simulink model "hexapod_LC"  (R2020b)
settings: Solver=VariableStepAuto  StartTime=0.0  StopTime=40.0  RelTol=1e-3
values from neighbouring files (symbols this model uses):
  goalPose = [13 13 0]    [Run_Sim_LC.m]
  N = size(waypoints, 1)    [interpolate_leg_waypoints.m]
  startPose = [2 2 0]    [Run_Sim_LC.m]
  Ts = 0.01    [Run_Sim_LC.m]
undefined symbols (not defined in the file or in its folder): Discrete, q, qd, Time, X, Y, Z
libraries: sm_lib x12, legs x8, nesl_utility x3, robotics_pg_exp_pack x2, ctrlSharedLib x1
settings Model: Creator=fciriell  LastModifiedBy=zach
settings ExplorerConfigSet: InternalSimMechanicsExplorerSettings="<ExplorerConfiguration><canonicalview>default</canonicalview><AnimationSetting><BasePlaybackSpeed>1.0</BasePlaybackSpeed><PlaybackSpeedFactor>1.0</PlaybackSpeedFactor></AnimationSetting><TilePanel><TileInfo><Tiles Columns=\"1\" Count=\"2\" Rows=\"2\"><Column Weight=\"1\"/><Row Weight=\"0.4993\"/><Row Weight=\"0.5007\"/><Tile Height=\"1\" Width=\"1\" X=\"0\" Y=\"0\"/><Tile Height=\"1\" Width=\"1\" X=\"0\" Y=\"1\"/></Tiles></TileInfo><SceneInfo><SceneViewer><BGColor><R>1</R><G>1</G><B>1</B></BGColor><Camera><DoPerspective>on</DoPerspective><Position><X>-4.35147948962821829e-06</X><Y>-4.89869399804638128</Y><Z>0.176731420553238427</Z></Position><Center><X>-4.35147948962821829e-06</X><Y>-1.26250265135058726</Y><Z>0.176731420553238427</Z></Center><Up><X>0</X><Y>-0</Y><Z>1</Z></Up><ViewLimDist>1</ViewLimDist><YLim>0.466307658154998583</YLim><XLim>1.59125758717581123</XLim></Camera></SceneViewer><SceneViewer><BGColor><R>1</R><G>1</G><B>1</B></BGColor><Camera><DoPerspective>off</DoPerspective><Position><X>-5.9945065800093289e-08</X><Y>-3.21515629578642415</Y><Z>0.0606596897011122405</Z></Position><Center><X>-5.9945065800093289e-08</X><Y>-1.26250000733898382</Y><Z>0.0606596897011122405</Z></Center><Up><X>-0</X><Y>0</Y><Z>1</Z></Up><ViewLimDist>1</ViewLimDist><YLim>0.993270539045333911</YLim><XLim>3.37947076894122489</XLim></Camera></SceneViewer></SceneInfo></TilePanel><MechEditorPanel><Cameras><Camera><Id>Camera1</Id><Value><Name>Camera1</Name><NativeCamera><PositionTrackingFeature>camera.F</PositionTrackingFeature><CenterTrackingFeature>One_link_chain_dynamic.to_WF</CenterTrackingFeature><UpVectorTrackingFeature>camera.F</UpVectorTrackingFeature><CenterTrackingOrigin>on</CenterTrackingOrigin><UpVectorTrackingDirection>+Z</UpVectorTrackingDirection></NativeCamera></Value></Camera></Cameras><GfxPanelCameraMap><MapElement CameraMLId=\"Camera1\" GfxPanelIndex=\"0\"/></GfxPanelCameraMap><VideoCreator><PlaybackSpeedRatio>1.0</PlaybackSpeedRatio><FrameRate>30</FrameRate><VideoFormat>Motion JPEG AVI</VideoFormat><FrameSize>auto</FrameSize></VideoCreator></MechEditorPanel></ExplorerConfiguration>"

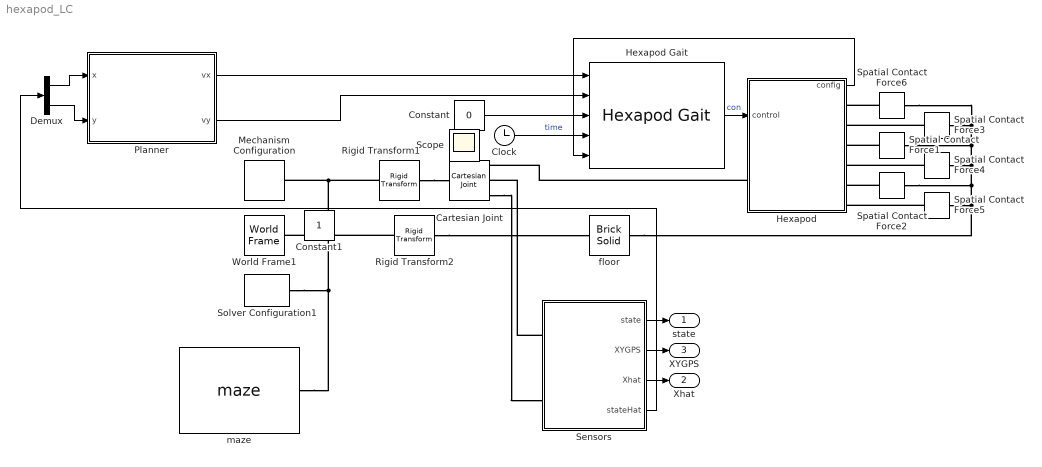
== system hexapod_LC ==
  Cartesian Joint : sm_lib/Joints/Cartesian Joint  JointMode=Normal  SenseConstraintForce=off  SenseConstraintForceX=off  SenseConstraintForceY=off  SenseConstraintForceZ=off  SenseConstraintTorque=off  SenseConstraintTorqueX=off  SenseConstraintTorqueY=off  SenseConstraintTorqueZ=off  SenseTotalForce=off  SenseTotalForceX=off  SenseTotalForceY=off  SenseTotalForceZ=off  SenseTotalTorque=off  SenseTotalTorqueX=off  SenseTotalTorqueY=off  SenseTotalTorqueZ=off  CompositeWrenchDir=FollowerOnBase  CompositeWrenchFrame=BaseFrame  PxEquilibriumPosition=0  PxEquilibriumPositionUnits=m  PxSpringStiffness=0  PxSpringStiffnessUnits=N/m  PxDampingCoefficient=0  PxDampingCoefficientUnits=N/(m/s)  PxTorqueActuationMode=NoTorque  PxMotionActuationMode=ComputedMotion  PxSensePosition=on  PxSenseVelocity=off  PxSenseAcceleration=off  PxSenseTorqueForce=off  PxSenseLowerLimitTorqueForce=off  PxSenseUpperLimitTorqueForce=off  PxLowerLimitSpecify=off  PxLowerLimitBound=-1  PxLowerLimitBoundUnits=m  PxLowerLimitStiffness=1e6  PxLowerLimitStiffnessUnits=N/m  PxLowerLimitDamping=1e3  PxLowerLimitDampingUnits=N/(m/s)  PxLowerLimitTransitionRegionWidth=1e-4  PxLowerLimitTransitionRegionWidthUnits=m  PxUpperLimitSpecify=off  PxUpperLimitBound=1  PxUpperLimitBoundUnits=m  PxUpperLimitStiffness=1e6  PxUpperLimitStiffnessUnits=N/m  PxUpperLimitDamping=1e3  PxUpperLimitDampingUnits=N/(m/s)  PxUpperLimitTransitionRegionWidth=1e-4  PxUpperLimitTransitionRegionWidthUnits=m  PxPositionTargetSpecify=on  PxPositionTargetPriority=High  PxPositionTargetValue=0  PxPositionTargetValueUnits=m  PxVelocityTargetSpecify=off  PxVelocityTargetPriority=High  PxVelocityTargetValue=0  PxVelocityTargetValueUnits=m/s  PyEquilibriumPosition=0  PyEquilibriumPositionUnits=m  PySpringStiffness=0  PySpringStiffnessUnits=N/m  PyDampingCoefficient=0  PyDampingCoefficientUnits=N/(m/s)  PyTorqueActuationMode=NoTorque  PyMotionActuationMode=ComputedMotion  PySensePosition=on  PySenseVelocity=off  PySenseAcceleration=off  PySenseTorqueForce=off  PySenseLowerLimitTorqueForce=off  PySenseUpperLimitTorqueForce=off  PyLowerLimitSpecify=off  PyLowerLimitBound=-1  PyLowerLimitBoundUnits=m  PyLowerLimitStiffness=1e6  PyLowerLimitStiffnessUnits=N/m  PyLowerLimitDamping=1e3  PyLowerLimitDampingUnits=N/(m/s)  PyLowerLimitTransitionRegionWidth=1e-4  PyLowerLimitTransitionRegionWidthUnits=m  PyUpperLimitSpecify=off  PyUpperLimitBound=1  PyUpperLimitBoundUnits=m  PyUpperLimitStiffness=1e6  PyUpperLimitStiffnessUnits=N/m  PyUpperLimitDamping=1e3  PyUpperLimitDampingUnits=N/(m/s)  PyUpperLimitTransitionRegionWidth=1e-4  PyUpperLimitTransitionRegionWidthUnits=m  PyPositionTargetSpecify=on  PyPositionTargetPriority=High  PyPositionTargetValue=0  PyPositionTargetValueUnits=m  PyVelocityTargetSpecify=off  PyVelocityTargetPriority=High  PyVelocityTargetValue=0  PyVelocityTargetValueUnits=m/s  PzEquilibriumPosition=0  PzEquilibriumPositionUnits=m  PzSpringStiffness=0  PzSpringStiffnessUnits=N/m  PzDampingCoefficient=0  PzDampingCoefficientUnits=N/(m/s)  PzTorqueActuationMode=NoTorque  PzMotionActuationMode=ComputedMotion  PzSensePosition=off  PzSenseVelocity=off  PzSenseAcceleration=off  PzSenseTorqueForce=off  PzSenseLowerLimitTorqueForce=off  PzSenseUpperLimitTorqueForce=off  PzLowerLimitSpecify=off  PzLowerLimitBound=-1  PzLowerLimitBoundUnits=m  PzLowerLimitStiffness=1e6  PzLowerLimitStiffnessUnits=N/m  PzLowerLimitDamping=1e3  PzLowerLimitDampingUnits=N/(m/s)  PzLowerLimitTransitionRegionWidth=1e-4  PzLowerLimitTransitionRegionWidthUnits=m  PzUpperLimitSpecify=off  PzUpperLimitBound=1  PzUpperLimitBoundUnits=m  PzUpperLimitStiffness=1e6  PzUpperLimitStiffnessUnits=N/m  PzUpperLimitDamping=1e3  PzUpperLimitDampingUnits=N/(m/s)  PzUpperLimitTransitionRegionWidth=1e-4  PzUpperLimitTransitionRegionWidthUnits=m  PzPositionTargetSpecify=on  PzPositionTargetPriority=High  PzPositionTargetValue=0.6  PzPositionTargetValueUnits=m  PzVelocityTargetSpecify=off  PzVelocityTargetPriority=High  PzVelocityTargetValue=0  PzVelocityTargetValueUnits=m/s
  Clock : Clock
  Constant : Constant  Value=0  SampleTime=-1
  Demux : Demux  Outputs=2
  Hexapod : Subsystem  AncestorBlock=legs/Hexapod  mask{leg_initial_config=[0; pi/8; 3*pi/8], leg_length_1=0.1, leg_length_2=0.4, leg_length_3=0.4, leg_radius=0.04, leg_mass_1=0.1, leg_mass_2=0.3, leg_mass_3=0.3, pos_kp=[40; 40; 40], pos_ki=[0; 0; 0], pos_kd=[4; 4; 4], body_radius=0.3, body_mass=0.2}
      mask prompts: leg_initial_config "Leg initial config"; leg_length_1 "Leg length 1"; leg_length_2 "Leg length 2"; leg_length_3 "Leg length 3"; leg_radius "Leg radius"; leg_mass_1 "Leg mass 1"; leg_mass_2 "Leg mass 2"; leg_mass_3 "Leg mass 3"; pos_kp "Position control kp"; pos_ki "Position control ki"; pos_kd "Position control kd"; body_radius "Body radius"; body_mass "Body mass"
  Hexapod Gait : legs/Hexapod Gait  beta=0.5  T=0.7  contact_start_config=[0; pi/8; 3*pi/8]  lifted_mid_theta2=-pi/2  lifted_mid_theta3=3*pi/4  body_radius=0.3  leg_length_1=0.1  leg_length_2=0.4  leg_length_3=0.4
      settings: SourceProductName=Legs
  Mechanism Configuration : sm_lib/Utilities/Mechanism Configuration  UniformGravity=Constant  GravityVector=[0 0 -9.80665]  GravityVectorUnits=m/s^2  GravityUnits=m/s^2  LinearizationDelta=0.001  JointModeTransitionNonlinearIterations=2
  Planner : Subsystem
  Rigid Transform1 : sm_lib/Frames and Transforms/Rigid Transform  TranslationMethod=Cartesian  TranslationStandardOffset=0  TranslationLengthUnit=m  TranslationStandardAxis=+Z  TranslationCartesianOffset=[2 2 0]  TranslationROffset=0  TranslationROffsetUnits=m  TranslationZOffset=0  TranslationZOffsetUnits=m  TranslationThetaOffset=0  TranslationThetaOffsetUnits=deg  RotationMethod=None  RotationAngleUnits=deg  RotationStandardAxis=+Z  RotationAngle=0.0  RotationArbitraryAxis=[0 0 1]  FollAlignAxisA=+X  BaseAlignAxisA=+Y  FollAlignAxisB=+Y  BaseAlignAxisB=+Z  RotationSequenceAxes=FollowerAxes  RotationSequence=XYX  RotationSequenceAngles=[0 0 0]  RotationSequenceAnglesUnits=deg  RotationMatrix=[1 0 0; 0 1 0; 0 0 1]
  Rigid Transform2 : sm_lib/Frames and Transforms/Rigid Transform  TranslationMethod=Cartesian  TranslationStandardOffset=0  TranslationLengthUnit=m  TranslationStandardAxis=+Z  TranslationCartesianOffset=[7.5 7.5 0]  TranslationROffset=0  TranslationROffsetUnits=m  TranslationZOffset=0  TranslationZOffsetUnits=m  TranslationThetaOffset=0  TranslationThetaOffsetUnits=deg  RotationMethod=None  RotationAngleUnits=deg  RotationStandardAxis=+Z  RotationAngle=0.0  RotationArbitraryAxis=[0 0 1]  FollAlignAxisA=+X  BaseAlignAxisA=+Y  FollAlignAxisB=+Y  BaseAlignAxisB=+Z  RotationSequenceAxes=FollowerAxes  RotationSequence=XYX  RotationSequenceAngles=[0 0 0]  RotationSequenceAnglesUnits=deg  RotationMatrix=[1 0 0; 0 1 0; 0 0 1]
  Sensors : Subsystem
  Solver Configuration1 : nesl_utility/Solver Configuration  PhysicalDomain=network_engine_domain  SubClassName=solver  LeftPortType=input  RightPortType=generic  Tones=[]  Harmonics=[]  SimulateNoise=off  Profile=off  UseLocalSampling=off  EnableSwitchedLinearOptims=on  FrequencyDomain=off  UseCCode=off  RelTol=0.001  AbsTol=1e-06  MinStep=1e-09  ToWorkspace=off  RevertToSquareIcSolve=off  NumHomotopyIterations=100  PhasorMode=off  PhasorModeNumHarmonics=1  DoDC=off  ResidualTolerance=1e-09  UseLocalSolver=off  LocalSolverChoice=NE_BACKWARD_EULER_ADVANCER  LocalSolverSampleTime=0.001  DoFixedCost=off  MaxNonlinIter=3  MaxModeIter=2  ComputeImpulses=off  ImpulseIterations=2  LinearAlgebra=auto  EquationFormulation=NE_TIME_EF  DelaysMemoryBudget=1024  AutomaticFiltering=on  FilteringTimeConstant=0.001  PartitionStorageMethod=AS_NEEDED  PartitionMemoryBudget=1024  PartitionMethod=ROBUST
  Spatial Contact Force{1..6} (6 alike) : sm_lib/Forces and Torques/Spatial Contact Force  CoefficientOfDynamicFriction=0.3  CoefficientOfStaticFriction=0.9  NormalDamping=1e3  NormalDampingUnits=N/(m/s)  NormalStiffness=1e6  NormalStiffnessUnits=N/m  FrictionalCriticalVelocity=1e-3  FrictionalCriticalVelocityUnits=m/s  ZeroCrossDetectContactStartAndEnd=off  SenseFrictionalForceMagnitude=off  SenseNormalForceMagnitude=off  SenseSeparationDistance=off  NormalTransitionRegionWidth=1e-4  NormalTransitionRegionWidthUnits=m  FrictionType=SmoothStickSlip
  World Frame1 : sm_lib/Frames and Transforms/World Frame
  floor : sm_lib/Body Elements/Brick Solid  GraphicAmbientColor=[0.15 0.15 0.15 1.0]  BasedOnType=Density  BrickDimensions=[20 20 0.5]  BrickDimensionUnits=m  CenterOfMass=[0 0 0]  CenterOfMassUnits=m  GraphicDiffuseColor=[0.5 0.5 0.5]  Density=1000  DensityUnits=kg/m^3  DoExposeReferenceFrame=off  GraphicEmissiveColor=[0.0 0.0 0.0 1.0]  ExportEntireGeometry=on  SerializedFrames=<Frames><Frame><Id>Frame1</Id><Value><Name>TF</Name><Origin><Source>GeometricFeature</Source><FeatureName>+z surface</FeatureName></Origin><PrimaryAxis><DefinedDirection>+Z</DefinedDirection><Source>ReferenceFrame</Source><SourceDirection>+Z</SourceDirection><FeatureName></FeatureName></PrimaryAxis><SecondaryAxis><DefinedDirection>+X</DefinedDirection><Source>ReferenceFrame</Source><SourceDirection>+X</SourceDirection><FeatureName></FeatureName></SecondaryAxis></Value></Frame></Frames>  MarkerShape=Sphere  MarkerSize=10  GraphicType=FromGeometry  InertiaType=CalculateFromGeometry  Mass=1  MassUnits=kg  MomentsOfInertia=[1 1 1]  MomentsOfInertiaUnits=kg*m^2  GraphicOpacity=0.5  ProductsOfInertia=[0 0 0]  ProductsOfInertiaUnits=kg*m^2  GraphicShininess=75  GraphicSpecularColor=[0.5 0.5 0.5 1.0]  GraphicVisPropType=SimpleVisualProperties
  maze : robotics_pg_exp_pack/Environments & Sensors/Simscape Multibody Environments/maze  map=maze  wall_height=0.5  resolution=res  branching=branching
      settings: SourceProductName=Robotics Playground Expansion Pack
  state : Outport
  Xhat : Outport  Port=2
  XYGPS : Outport  Port=3
  Constant1 : Constant  IOType=siggen
  Scope : Scope
  wires:
  Hexapod Gait/1 -> Hexapod/1(control)  "con"
  Hexapod/1(config) -> Hexapod Gait/5
  Constant/1 -> Hexapod Gait/3
  Clock/1 -> Hexapod Gait/4  "time"
  Sensors/1(state) -> state/1
  Sensors/2(XYGPS) -> XYGPS/1
  Sensors/3(Xhat) -> Xhat/1
  Sensors/4(stateHat) -> Demux/1
  Demux/1 -> Planner/1(x)
  Demux/2 -> Planner/2(y)
  Planner/2(vy) -> Hexapod Gait/2
  Planner/1(vx) -> Hexapod Gait/1
  connections:
  Solver Configuration1/RConn1 -- maze/RConn1 -- Rigid Transform2/LConn1 -- Rigid Transform1/LConn1 -- Mechanism Configuration/RConn1 -- World Frame1/RConn1
  Hexapod/LConn1 -- Cartesian Joint/RConn1
  floor/RConn1 -- Spatial Contact Force5/LConn1 -- Spatial Contact Force2/LConn1 -- Spatial Contact Force4/LConn1 -- Spatial Contact Force1/LConn1 -- Spatial Contact Force3/LConn1 -- Spatial Contact Force6/LConn1
  Spatial Contact Force6/RConn1 -- Hexapod/RConn1
  Spatial Contact Force3/RConn1 -- Hexapod/RConn2
  Spatial Contact Force4/RConn1 -- Hexapod/RConn4
  Spatial Contact Force5/RConn1 -- Hexapod/RConn6
  Spatial Contact Force2/RConn1 -- Hexapod/RConn5
  Spatial Contact Force1/RConn1 -- Hexapod/RConn3
  Rigid Transform2/RConn1 -- floor/LConn1
  Rigid Transform1/RConn1 -- Cartesian Joint/LConn1
  Sensors/LConn1 -- Cartesian Joint/RConn2
  Cartesian Joint/RConn3 -- Sensors/LConn2

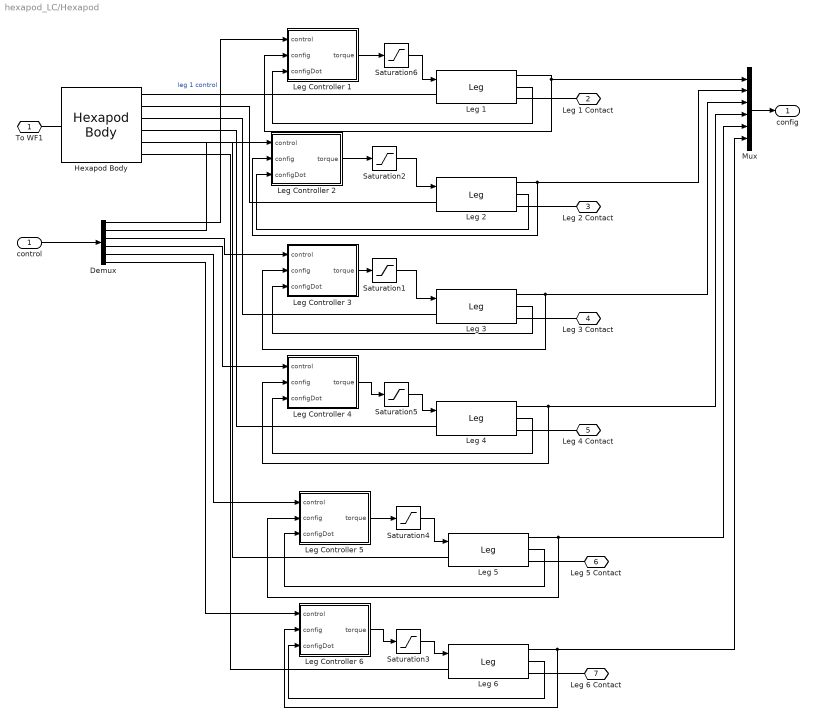
== system hexapod_LC/Hexapod ==
  control : Inport
  Demux : Demux  Outputs=6
  Hexapod Body : legs/Hexapod Body  radius=body_radius  height=leg_radius*2  leg_radius=leg_radius  mass=body_mass
      settings: SourceProductName=Legs
  Leg {1..6} (6 alike) : legs/Leg  length_1=leg_length_1  length_2=leg_length_2  length_3=leg_length_3  radius=leg_radius  mass_1=leg_mass_1  mass_2=leg_mass_2  mass_3=leg_mass_3  initial_config=leg_initial_config
      settings: SourceProductName=Legs
  Leg Controller 1 : Subsystem  AncestorBlock=legs/Leg Controller  mask{pos_kp=pos_kp, pos_ki=pos_ki, pos_kd=pos_kd, initial_config=leg_initial_config}
      mask prompts: pos_kp "Position control kp"; pos_ki "Position control ki"; pos_kd "Position control kd"; initial_config "Initial config"
  Leg Controller 2 : Subsystem  AncestorBlock=legs/Leg Controller  mask{pos_kp=pos_kp, pos_ki=pos_ki, pos_kd=pos_kd, initial_config=leg_initial_config}
      mask prompts: pos_kp "Position control kp"; pos_ki "Position control ki"; pos_kd "Position control kd"; initial_config "Initial config"
  Leg Controller 3 : Subsystem  AncestorBlock=legs/Leg Controller  mask{pos_kp=pos_kp, pos_ki=pos_ki, pos_kd=pos_kd, initial_config=leg_initial_config}
      mask prompts: pos_kp "Position control kp"; pos_ki "Position control ki"; pos_kd "Position control kd"; initial_config "Initial config"
  Leg Controller 4 : Subsystem  AncestorBlock=legs/Leg Controller  mask{pos_kp=pos_kp, pos_ki=pos_ki, pos_kd=pos_kd, initial_config=leg_initial_config}
      mask prompts: pos_kp "Position control kp"; pos_ki "Position control ki"; pos_kd "Position control kd"; initial_config "Initial config"
  Leg Controller 5 : Subsystem  AncestorBlock=legs/Leg Controller  mask{pos_kp=pos_kp, pos_ki=pos_ki, pos_kd=pos_kd, initial_config=leg_initial_config}
      mask prompts: pos_kp "Position control kp"; pos_ki "Position control ki"; pos_kd "Position control kd"; initial_config "Initial config"
  Leg Controller 6 : Subsystem  AncestorBlock=legs/Leg Controller  mask{pos_kp=pos_kp, pos_ki=pos_ki, pos_kd=pos_kd, initial_config=leg_initial_config}
      mask prompts: pos_kp "Position control kp"; pos_ki "Position control ki"; pos_kd "Position control kd"; initial_config "Initial config"
  Mux : Mux  Inputs=6
  Saturation{1..6} (6 alike) : Saturate  UpperLimit=20  LowerLimit=-20
  To WF1 : PMIOPort  Side=Left
  Leg 1 Contact : PMIOPort  Port=2  Side=Right
  Leg 2 Contact : PMIOPort  Port=3  Side=Right
  Leg 3 Contact : PMIOPort  Port=4  Side=Right
  Leg 4 Contact : PMIOPort  Port=5  Side=Right
  Leg 5 Contact : PMIOPort  Port=6  Side=Right
  Leg 6 Contact : PMIOPort  Port=7  Side=Right
  config : Outport
  wires:
  Mux/1 -> config/1
  Demux/6 -> Leg Controller 6/1(control)
  control/1 -> Demux/1
  Leg 5/1 -> Mux/5, Leg Controller 5/2(config)
  Leg 5/2 -> Leg Controller 5/3(configDot)
  Leg 6/2 -> Leg Controller 6/3(configDot)
  Leg Controller 6/1(torque) -> Saturation3/1
  Demux/5 -> Leg Controller 5/1(control)
  Leg 6/1 -> Mux/6, Leg Controller 6/2(config)
  Leg Controller 5/1(torque) -> Saturation4/1
  Leg Controller 2/1(torque) -> Saturation2/1
  Leg Controller 3/1(torque) -> Saturation1/1
  Leg 1/2 -> Leg Controller 1/3(configDot)
  Leg 3/1 -> Mux/3, Leg Controller 3/2(config)
  Leg 4/2 -> Leg Controller 4/3(configDot)
  Leg Controller 4/1(torque) -> Saturation5/1
  Leg 4/1 -> Mux/4, Leg Controller 4/2(config)
  Demux/3 -> Leg Controller 3/1(control)
  Demux/1 -> Leg Controller 1/1(control)  "leg 1 control"
  Demux/4 -> Leg Controller 4/1(control)
  Leg 3/2 -> Leg Controller 3/3(configDot)
  Demux/2 -> Leg Controller 2/1(control)
  Leg 1/1 -> Mux/1, Leg Controller 1/2(config)
  Leg 2/1 -> Mux/2, Leg Controller 2/2(config)
  Leg 2/2 -> Leg Controller 2/3(configDot)
  Leg Controller 1/1(torque) -> Saturation6/1
  Saturation6/1 -> Leg 1/1
  Saturation2/1 -> Leg 2/1
  Saturation1/1 -> Leg 3/1
  Saturation5/1 -> Leg 4/1
  Saturation4/1 -> Leg 5/1
  Saturation3/1 -> Leg 6/1
  connections:
  Leg 5/LConn1 -- Hexapod Body/RConn5
  Leg 6/RConn1 -- Leg 6 Contact/RConn1
  Leg 5/RConn1 -- Leg 5 Contact/RConn1
  Leg 6/LConn1 -- Hexapod Body/RConn6
  Hexapod Body/LConn1 -- To WF1/RConn1
  Leg 3/RConn1 -- Leg 3 Contact/RConn1
  Leg 4/RConn1 -- Leg 4 Contact/RConn1
  Leg 2/RConn1 -- Leg 2 Contact/RConn1
  Leg 4/LConn1 -- Hexapod Body/RConn4
  Leg 1/LConn1 -- Hexapod Body/RConn1
  Leg 2/LConn1 -- Hexapod Body/RConn2
  Leg 3/LConn1 -- Hexapod Body/RConn3
  Leg 1 Contact/RConn1 -- Leg 1/RConn1

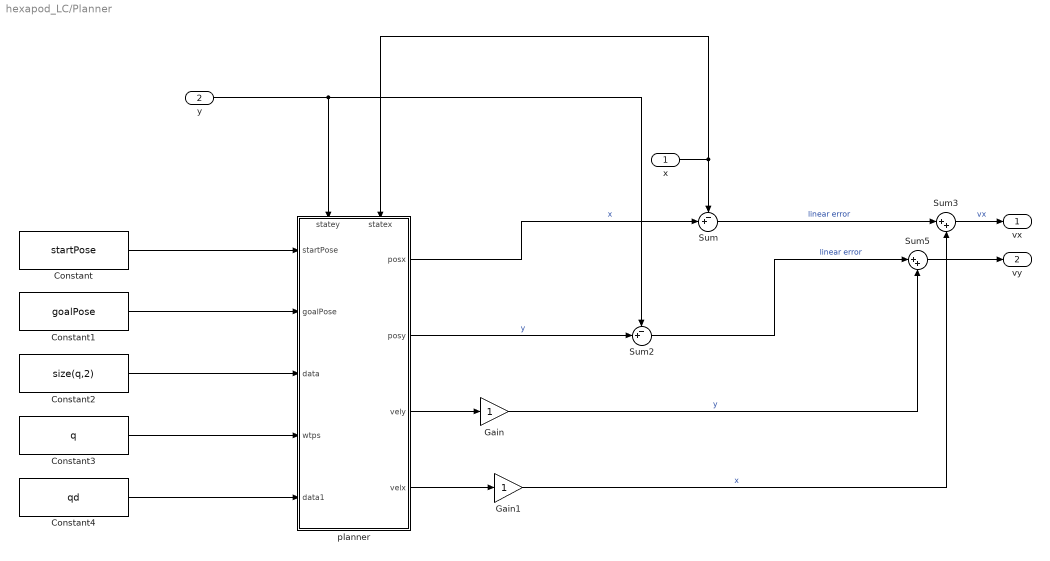
== system hexapod_LC/Planner ==
  x : Inport
  y : Inport  Port=2
  Constant : Constant  Value=startPose  SampleTime=Ts
  Constant1 : Constant  Value=goalPose  SampleTime=Ts
  Constant2 : Constant  Value=size(q,2)  SampleTime=Ts
  Constant3 : Constant  Value=q  SampleTime=Ts
  Constant4 : Constant  Value=qd  SampleTime=Ts
  Gain : Gain
  Gain1 : Gain
  Sum : Sum  Inputs=-+|
  Sum2 : Sum  Inputs=-+|
  Sum3 : Sum  Inputs=|++
  Sum5 : Sum  Inputs=|++
  planner : Stateflow chart  TreatAsAtomicUnit=on
      settings: PortSchema="{\"entries\":[{\"content\":{\"sides\":[{\"content\":{\"connectorIds\":[\"In1\",\"In2\",\"In3\",\"In5\",\"In4\"]},\"type\":\"ConnectorPlacement.EquallySpacedRectSide\",\"uuid\":\"da1c7cfa-1c14-4526-9179-9c171806de56\"},{\"content\":{\"connectorIds\":[\"Out4\",\"Out3\",\"Out1\",\"Out2\"],\"side\":\"RIGHT\"},\"type\":\"ConnectorPlacement.EquallySpacedRectSide\",\"uuid\":\"2bfdc814-d91f-4ce3-acc2-08fb6905f934\"},{\"content\":{\"connectorIds\":[\"In7\",\"In6\"],\"side\":\"TOP\"},\"type\":\"ConnectorPlacement.EquallySpacedRectSide\",\"uuid\":\"554321fd-f0cc-4939-8c5c-38ba428d6ed5\"},{\"content\":{\"connectorIds\":[],\"side\":\"HIDDEN\"},\"type\":\"ConnectorPlacement.EquallySpacedRectSide\",\"uuid\":\"12925c00-27c4-4cf0-b4a8-d9f38fa42e90\"}]},\"type\":\"ConnectorPlacement.EquallySpacedConnector\",\"uuid\":\"448e04cb-c50a-4a7a-8276-726a8daf06ad\"}],\"packageUris\":[\"http://schema.mathworks.com/mf0/Connector/R2020b\"],\"version\":\"1.0\"}"
  vx : Outport
  vy : Outport  Port=2
  wires:
  planner/4(posx) -> Sum/2  "x"
  Sum/1 -> Sum3/1  "linear error"
  planner/3(posy) -> Sum2/2  "y"
  Sum2/1 -> Sum5/1  "linear error"
  planner/2(velx) -> Gain1/1
  Constant1/1 -> planner/2(goalPose)
  planner/1(vely) -> Gain/1
  Constant/1 -> planner/1(startPose)
  Gain1/1 -> Sum3/2  "x"
  Gain/1 -> Sum5/2  "y"
  Constant3/1 -> planner/5(wtps)
  Constant4/1 -> planner/4(data1)
  y/1 -> Sum2/1, planner/7(statey)
  x/1 -> planner/6(statex), Sum/1
  Sum3/1 -> vx/1  "vx"
  Constant2/1 -> planner/3(data)
  Sum5/1 -> vy/1

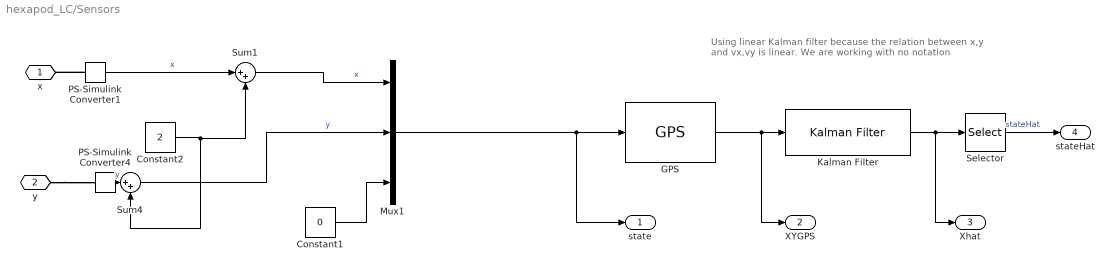
== system hexapod_LC/Sensors ==
  note: Using linear Kalman filter because the relation between x,y and vx,vy is linear. We are working with no notation
  Constant1 : Constant  Value=0  SampleTime=Ts
  Constant2 : Constant  Value=2
  "GPS " : robotics_pg_exp_pack/Environments & Sensors/GPS  xNoisePower=0.05  yNoisePower=0.05  Ts=Ts
      settings: SourceProductName=Robotics Playground Expansion Pack
  "Kalman Filter " : ctrlSharedLib/Kalman Filter  TimeDomain=Discrete-Time  UseCurrentEstimator=on  ModelSource=Individual A, B, C, D matrices  ModelSourceVariable=sys  A=[1 0 Ts 0; 0 1 0 Ts; 0 0 1 0; 0 0 0 1]  B=eye(2)  C=[1 0 0 0; 0 1 0 0]  D=zeros(2)  NumberOfStates=2  NumberOfInputs=2  NumberOfOutputs=2  InitialEstimateSource=Dialog  X0=0  P0=1e-3  UseK=off  UseGH=on  NumberOfProcessNoiseInputs=2  G=[Ts/2 0; 0 Ts/2; 1 0; 0 1]  TimeInvariantG=on  H=0  TimeInvariantH=on  Q=0.12  TimeInvariantQ=on  R=0.08  TimeInvariantR=on  N=0  TimeInvariantN=on  AddInputPort=off  AddEnablePort=off  OutputEstimatedY=off  OutputP=off  Ts=Ts
  Mux1 : Mux  Inputs=3
  PS-Simulink Converter1 : nesl_utility/PS-Simulink Converter  PhysicalDomain=network_engine_domain  SubClassName=ps_output  LeftPortType=input  RightPortType=output  PseudoPeriodic=off  Frequencies=[]  Unit=1  AffineConversion=off
  PS-Simulink Converter4 : nesl_utility/PS-Simulink Converter  PhysicalDomain=network_engine_domain  SubClassName=ps_output  LeftPortType=input  RightPortType=output  PseudoPeriodic=off  Frequencies=[]  Unit=1  AffineConversion=off
  Selector : Selector  InputPortWidth=4  IndexOptions=Index vector (dialog)  Indices=[1 2]  OutputSizes=1
  Sum1 : Sum  Inputs=|++
  Sum4 : Sum  Inputs=|++
  x : PMIOPort  Side=Left
  y : PMIOPort  Port=2  Side=Left
  state : Outport
  XYGPS : Outport  Port=2
  Xhat : Outport  Port=3
  stateHat : Outport  Port=4
  wires:
  Constant2/1 -> Sum4/2, Sum1/2
  "GPS "/1 -> "Kalman Filter "/1, XYGPS/1
  PS-Simulink Converter1/1 -> Sum1/1  "x"
  Mux1/1 -> "GPS "/1, state/1
  Selector/1 -> stateHat/1  "stateHat"
  Sum4/1 -> Mux1/2  "y"
  PS-Simulink Converter4/1 -> Sum4/1  "y"
  Sum1/1 -> Mux1/1  "x"
  "Kalman Filter "/1 -> Selector/1, Xhat/1
  Constant1/1 -> Mux1/3
  connections:
  PS-Simulink Converter1/LConn1 -- x/RConn1
  y/RConn1 -- PS-Simulink Converter4/LConn1

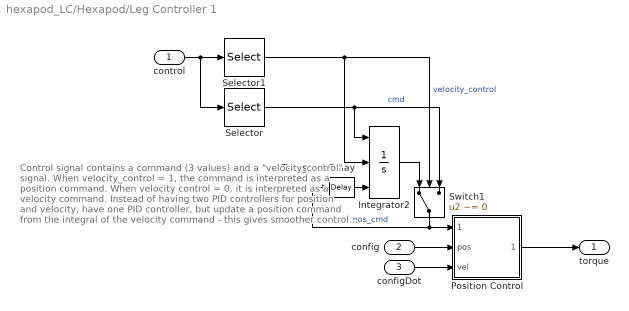
== system hexapod_LC/Hexapod/Leg Controller 1 ==
  note: Control signal contains a command (3 values)
      | and a "velocity_control" signal.
      |
      | When velocity_control = 1, the command is interpreted
      | as a position command. When velocity control = 0, it is
      | interpreted as a velocity command.
      |
      | Instead of having two PID controllers for position and velocity,
      | have one PID controller, but update a position command from
      | the integral of the velocity command - this gives smoother
      | control and is better at keeping a joint at a fixed angle when it
      | should have zero velocity.
      |
      | The integrator for the velocity command is reset to the last position
      | command when the velocity_control signal goes high. The easiest
      | way to do this is to add a small delay on the pos_cmd signal.
      | The delay can also accept an initial value, which is set to the initial
      | joint values.
  control : Inport
  config : Inport  Port=2
  configDot : Inport  Port=3
  Integrator2 : Integrator  ExternalReset=rising  InitialConditionSource=external
  Position Control : Subsystem
  Selector : Selector  InputPortWidth=4  IndexOptions=Index vector (dialog)  Indices=[1 2 3]  OutputSizes=1
  Selector1 : Selector  InputPortWidth=4  IndexOptions=Index vector (dialog)  Indices=[4]  OutputSizes=1
  Switch1 : Switch  Criteria=u2 ~= 0
  Transport Delay : TransportDelay  DelayTime=0.01  InitialOutput=initial_config
  torque : Outport
  wires:
  Transport Delay/1 -> Integrator2/3
  Switch1/1 -> Position Control/1(pos_cmd), Transport Delay/1  "pos_cmd"
  Selector/1 -> Switch1/3, Integrator2/1  "cmd"
  Integrator2/1 -> Switch1/1
  Selector1/1 -> Switch1/2, Integrator2/2  "velocity_control"
  Position Control/1(torque) -> torque/1
  configDot/1 -> Position Control/3(vel)
  config/1 -> Position Control/2(pos)
  control/1 -> Selector/1, Selector1/1

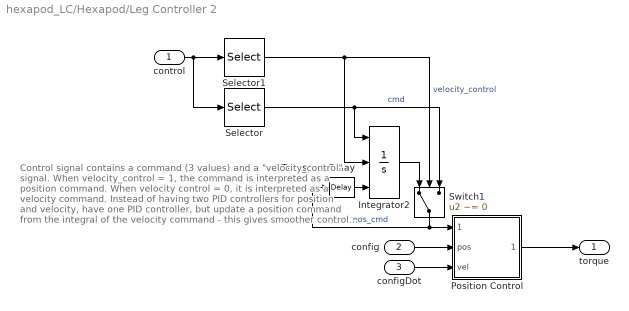
== system hexapod_LC/Hexapod/Leg Controller 2 ==
  note: Control signal contains a command (3 values)
      | and a "velocity_control" signal.
      |
      | When velocity_control = 1, the command is interpreted
      | as a position command. When velocity control = 0, it is
      | interpreted as a velocity command.
      |
      | Instead of having two PID controllers for position and velocity,
      | have one PID controller, but update a position command from
      | the integral of the velocity command - this gives smoother
      | control and is better at keeping a joint at a fixed angle when it
      | should have zero velocity.
      |
      | The integrator for the velocity command is reset to the last position
      | command when the velocity_control signal goes high. The easiest
      | way to do this is to add a small delay on the pos_cmd signal.
      | The delay can also accept an initial value, which is set to the initial
      | joint values.
  control : Inport
  config : Inport  Port=2
  configDot : Inport  Port=3
  Integrator2 : Integrator  ExternalReset=rising  InitialConditionSource=external
  Position Control : Subsystem
  Selector : Selector  InputPortWidth=4  IndexOptions=Index vector (dialog)  Indices=[1 2 3]  OutputSizes=1
  Selector1 : Selector  InputPortWidth=4  IndexOptions=Index vector (dialog)  Indices=[4]  OutputSizes=1
  Switch1 : Switch  Criteria=u2 ~= 0
  Transport Delay : TransportDelay  DelayTime=0.01  InitialOutput=initial_config
  torque : Outport
  wires:
  Transport Delay/1 -> Integrator2/3
  Switch1/1 -> Position Control/1(pos_cmd), Transport Delay/1  "pos_cmd"
  Selector/1 -> Switch1/3, Integrator2/1  "cmd"
  Integrator2/1 -> Switch1/1
  Selector1/1 -> Switch1/2, Integrator2/2  "velocity_control"
  Position Control/1(torque) -> torque/1
  configDot/1 -> Position Control/3(vel)
  config/1 -> Position Control/2(pos)
  control/1 -> Selector/1, Selector1/1

== system hexapod_LC/Hexapod/Leg Controller 3 ==
  note: Control signal contains a command (3 values)
      | and a "velocity_control" signal.
      |
      | When velocity_control = 1, the command is interpreted
      | as a position command. When velocity control = 0, it is
      | interpreted as a velocity command.
      |
      | Instead of having two PID controllers for position and velocity,
      | have one PID controller, but update a position command from
      | the integral of the velocity command - this gives smoother
      | control and is better at keeping a joint at a fixed angle when it
      | should have zero velocity.
      |
      | The integrator for the velocity command is reset to the last position
      | command when the velocity_control signal goes high. The easiest
      | way to do this is to add a small delay on the pos_cmd signal.
      | The delay can also accept an initial value, which is set to the initial
      | joint values.
  control : Inport
  config : Inport  Port=2
  configDot : Inport  Port=3
  Integrator2 : Integrator  ExternalReset=rising  InitialConditionSource=external
  Position Control : Subsystem
  Selector : Selector  InputPortWidth=4  IndexOptions=Index vector (dialog)  Indices=[1 2 3]  OutputSizes=1
  Selector1 : Selector  InputPortWidth=4  IndexOptions=Index vector (dialog)  Indices=[4]  OutputSizes=1
  Switch1 : Switch  Criteria=u2 ~= 0
  Transport Delay : TransportDelay  DelayTime=0.01  InitialOutput=initial_config
  torque : Outport
  wires:
  Transport Delay/1 -> Integrator2/3
  Switch1/1 -> Position Control/1(pos_cmd), Transport Delay/1  "pos_cmd"
  Selector/1 -> Switch1/3, Integrator2/1  "cmd"
  Integrator2/1 -> Switch1/1
  Selector1/1 -> Switch1/2, Integrator2/2  "velocity_control"
  Position Control/1(torque) -> torque/1
  configDot/1 -> Position Control/3(vel)
  config/1 -> Position Control/2(pos)
  control/1 -> Selector/1, Selector1/1

== system hexapod_LC/Hexapod/Leg Controller 4 ==
  note: Control signal contains a command (3 values)
      | and a "velocity_control" signal.
      |
      | When velocity_control = 1, the command is interpreted
      | as a position command. When velocity control = 0, it is
      | interpreted as a velocity command.
      |
      | Instead of having two PID controllers for position and velocity,
      | have one PID controller, but update a position command from
      | the integral of the velocity command - this gives smoother
      | control and is better at keeping a joint at a fixed angle when it
      | should have zero velocity.
      |
      | The integrator for the velocity command is reset to the last position
      | command when the velocity_control signal goes high. The easiest
      | way to do this is to add a small delay on the pos_cmd signal.
      | The delay can also accept an initial value, which is set to the initial
      | joint values.
  control : Inport
  config : Inport  Port=2
  configDot : Inport  Port=3
  Integrator2 : Integrator  ExternalReset=rising  InitialConditionSource=external
  Position Control : Subsystem
  Selector : Selector  InputPortWidth=4  IndexOptions=Index vector (dialog)  Indices=[1 2 3]  OutputSizes=1
  Selector1 : Selector  InputPortWidth=4  IndexOptions=Index vector (dialog)  Indices=[4]  OutputSizes=1
  Switch1 : Switch  Criteria=u2 ~= 0
  Transport Delay : TransportDelay  DelayTime=0.01  InitialOutput=initial_config
  torque : Outport
  wires:
  Transport Delay/1 -> Integrator2/3
  Switch1/1 -> Position Control/1(pos_cmd), Transport Delay/1  "pos_cmd"
  Selector/1 -> Switch1/3, Integrator2/1  "cmd"
  Integrator2/1 -> Switch1/1
  Selector1/1 -> Switch1/2, Integrator2/2  "velocity_control"
  Position Control/1(torque) -> torque/1
  configDot/1 -> Position Control/3(vel)
  config/1 -> Position Control/2(pos)
  control/1 -> Selector/1, Selector1/1

== system hexapod_LC/Hexapod/Leg Controller 5 ==
  note: Control signal contains a command (3 values)
      | and a "velocity_control" signal.
      |
      | When velocity_control = 1, the command is interpreted
      | as a position command. When velocity control = 0, it is
      | interpreted as a velocity command.
      |
      | Instead of having two PID controllers for position and velocity,
      | have one PID controller, but update a position command from
      | the integral of the velocity command - this gives smoother
      | control and is better at keeping a joint at a fixed angle when it
      | should have zero velocity.
      |
      | The integrator for the velocity command is reset to the last position
      | command when the velocity_control signal goes high. The easiest
      | way to do this is to add a small delay on the pos_cmd signal.
      | The delay can also accept an initial value, which is set to the initial
      | joint values.
  control : Inport
  config : Inport  Port=2
  configDot : Inport  Port=3
  Integrator2 : Integrator  ExternalReset=rising  InitialConditionSource=external
  Position Control : Subsystem
  Selector : Selector  InputPortWidth=4  IndexOptions=Index vector (dialog)  Indices=[1 2 3]  OutputSizes=1
  Selector1 : Selector  InputPortWidth=4  IndexOptions=Index vector (dialog)  Indices=[4]  OutputSizes=1
  Switch1 : Switch  Criteria=u2 ~= 0
  Transport Delay : TransportDelay  DelayTime=0.01  InitialOutput=initial_config
  torque : Outport
  wires:
  Transport Delay/1 -> Integrator2/3
  Switch1/1 -> Position Control/1(pos_cmd), Transport Delay/1  "pos_cmd"
  Selector/1 -> Switch1/3, Integrator2/1  "cmd"
  Integrator2/1 -> Switch1/1
  Selector1/1 -> Switch1/2, Integrator2/2  "velocity_control"
  Position Control/1(torque) -> torque/1
  configDot/1 -> Position Control/3(vel)
  config/1 -> Position Control/2(pos)
  control/1 -> Selector1/1, Selector/1

== system hexapod_LC/Hexapod/Leg Controller 6 ==
  note: Control signal contains a command (3 values)
      | and a "velocity_control" signal.
      |
      | When velocity_control = 1, the command is interpreted
      | as a position command. When velocity control = 0, it is
      | interpreted as a velocity command.
      |
      | Instead of having two PID controllers for position and velocity,
      | have one PID controller, but update a position command from
      | the integral of the velocity command - this gives smoother
      | control and is better at keeping a joint at a fixed angle when it
      | should have zero velocity.
      |
      | The integrator for the velocity command is reset to the last position
      | command when the velocity_control signal goes high. The easiest
      | way to do this is to add a small delay on the pos_cmd signal.
      | The delay can also accept an initial value, which is set to the initial
      | joint values.
  control : Inport
  config : Inport  Port=2
  configDot : Inport  Port=3
  Integrator2 : Integrator  ExternalReset=rising  InitialConditionSource=external
  Position Control : Subsystem
  Selector : Selector  InputPortWidth=4  IndexOptions=Index vector (dialog)  Indices=[1 2 3]  OutputSizes=1
  Selector1 : Selector  InputPortWidth=4  IndexOptions=Index vector (dialog)  Indices=[4]  OutputSizes=1
  Switch1 : Switch  Criteria=u2 ~= 0
  Transport Delay : TransportDelay  DelayTime=0.01  InitialOutput=initial_config
  torque : Outport
  wires:
  Transport Delay/1 -> Integrator2/3
  Switch1/1 -> Position Control/1(pos_cmd), Transport Delay/1  "pos_cmd"
  Selector/1 -> Switch1/3, Integrator2/1  "cmd"
  Integrator2/1 -> Switch1/1
  Selector1/1 -> Switch1/2, Integrator2/2  "velocity_control"
  Position Control/1(torque) -> torque/1
  configDot/1 -> Position Control/3(vel)
  config/1 -> Position Control/2(pos)
  control/1 -> Selector1/1, Selector/1

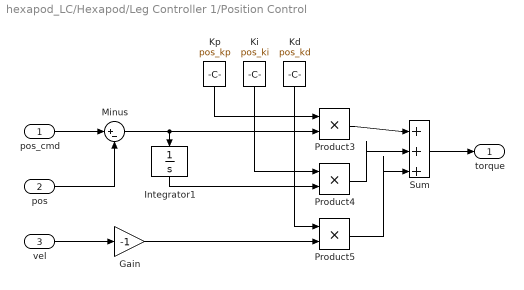
== system hexapod_LC/Hexapod/Leg Controller 1/Position Control ==
  pos_cmd : Inport
  pos : Inport  Port=2
  vel : Inport  Port=3
  Gain : Gain  Gain=-1
  Integrator1 : Integrator
  Kd : Constant  Value=pos_kd
  Ki : Constant  Value=pos_ki
  Kp : Constant  Value=pos_kp
  Minus : Sum  Inputs=|+-
  Product3 : Product
  Product4 : Product
  Product5 : Product
  Sum : Sum  Inputs=+++|
  torque : Outport
  wires:
  pos_cmd/1 -> Minus/1
  vel/1 -> Gain/1
  Gain/1 -> Product5/2
  Sum/1 -> torque/1
  Product3/1 -> Sum/1
  Kd/1 -> Product5/1
  Minus/1 -> Integrator1/1, Product3/2
  pos/1 -> Minus/2
  Integrator1/1 -> Product4/2
  Kp/1 -> Product3/1
  Ki/1 -> Product4/1
  Product5/1 -> Sum/3
  Product4/1 -> Sum/2

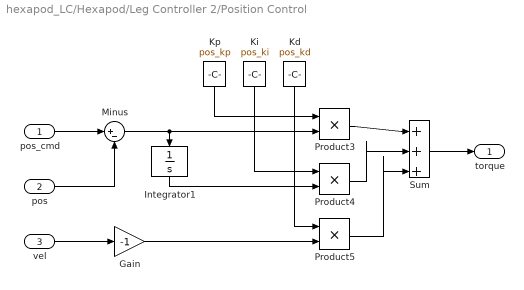
== system hexapod_LC/Hexapod/Leg Controller 2/Position Control ==
  pos_cmd : Inport
  pos : Inport  Port=2
  vel : Inport  Port=3
  Gain : Gain  Gain=-1
  Integrator1 : Integrator
  Kd : Constant  Value=pos_kd
  Ki : Constant  Value=pos_ki
  Kp : Constant  Value=pos_kp
  Minus : Sum  Inputs=|+-
  Product3 : Product
  Product4 : Product
  Product5 : Product
  Sum : Sum  Inputs=+++|
  torque : Outport
  wires:
  pos_cmd/1 -> Minus/1
  vel/1 -> Gain/1
  Gain/1 -> Product5/2
  Sum/1 -> torque/1
  Product3/1 -> Sum/1
  Kd/1 -> Product5/1
  Minus/1 -> Integrator1/1, Product3/2
  pos/1 -> Minus/2
  Integrator1/1 -> Product4/2
  Kp/1 -> Product3/1
  Ki/1 -> Product4/1
  Product5/1 -> Sum/3
  Product4/1 -> Sum/2

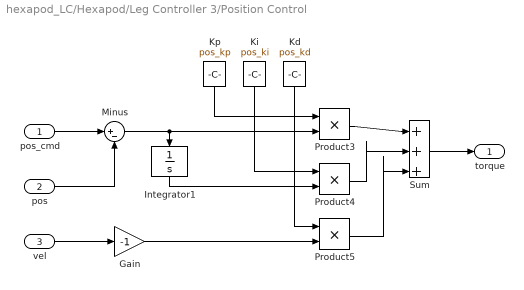
== system hexapod_LC/Hexapod/Leg Controller 3/Position Control ==
  pos_cmd : Inport
  pos : Inport  Port=2
  vel : Inport  Port=3
  Gain : Gain  Gain=-1
  Integrator1 : Integrator
  Kd : Constant  Value=pos_kd
  Ki : Constant  Value=pos_ki
  Kp : Constant  Value=pos_kp
  Minus : Sum  Inputs=|+-
  Product3 : Product
  Product4 : Product
  Product5 : Product
  Sum : Sum  Inputs=+++|
  torque : Outport
  wires:
  pos_cmd/1 -> Minus/1
  vel/1 -> Gain/1
  Gain/1 -> Product5/2
  Sum/1 -> torque/1
  Product3/1 -> Sum/1
  Kd/1 -> Product5/1
  Minus/1 -> Integrator1/1, Product3/2
  pos/1 -> Minus/2
  Integrator1/1 -> Product4/2
  Kp/1 -> Product3/1
  Ki/1 -> Product4/1
  Product5/1 -> Sum/3
  Product4/1 -> Sum/2

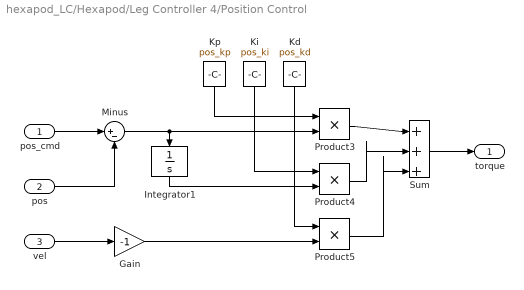
== system hexapod_LC/Hexapod/Leg Controller 4/Position Control ==
  pos_cmd : Inport
  pos : Inport  Port=2
  vel : Inport  Port=3
  Gain : Gain  Gain=-1
  Integrator1 : Integrator
  Kd : Constant  Value=pos_kd
  Ki : Constant  Value=pos_ki
  Kp : Constant  Value=pos_kp
  Minus : Sum  Inputs=|+-
  Product3 : Product
  Product4 : Product
  Product5 : Product
  Sum : Sum  Inputs=+++|
  torque : Outport
  wires:
  pos_cmd/1 -> Minus/1
  vel/1 -> Gain/1
  Gain/1 -> Product5/2
  Sum/1 -> torque/1
  Product3/1 -> Sum/1
  Kd/1 -> Product5/1
  Minus/1 -> Integrator1/1, Product3/2
  pos/1 -> Minus/2
  Integrator1/1 -> Product4/2
  Kp/1 -> Product3/1
  Ki/1 -> Product4/1
  Product5/1 -> Sum/3
  Product4/1 -> Sum/2

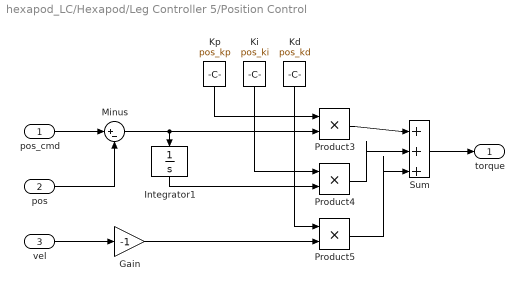
== system hexapod_LC/Hexapod/Leg Controller 5/Position Control ==
  pos_cmd : Inport
  pos : Inport  Port=2
  vel : Inport  Port=3
  Gain : Gain  Gain=-1
  Integrator1 : Integrator
  Kd : Constant  Value=pos_kd
  Ki : Constant  Value=pos_ki
  Kp : Constant  Value=pos_kp
  Minus : Sum  Inputs=|+-
  Product3 : Product
  Product4 : Product
  Product5 : Product
  Sum : Sum  Inputs=+++|
  torque : Outport
  wires:
  pos_cmd/1 -> Minus/1
  vel/1 -> Gain/1
  Gain/1 -> Product5/2
  Sum/1 -> torque/1
  Product3/1 -> Sum/1
  Kd/1 -> Product5/1
  Minus/1 -> Integrator1/1, Product3/2
  pos/1 -> Minus/2
  Integrator1/1 -> Product4/2
  Kp/1 -> Product3/1
  Ki/1 -> Product4/1
  Product5/1 -> Sum/3
  Product4/1 -> Sum/2

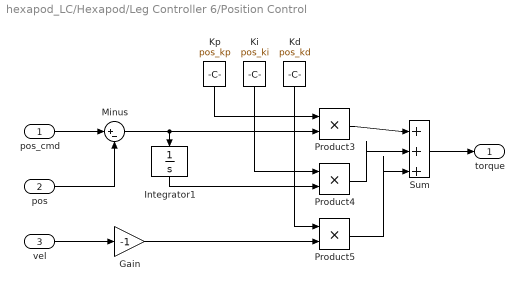
== system hexapod_LC/Hexapod/Leg Controller 6/Position Control ==
  pos_cmd : Inport
  pos : Inport  Port=2
  vel : Inport  Port=3
  Gain : Gain  Gain=-1
  Integrator1 : Integrator
  Kd : Constant  Value=pos_kd
  Ki : Constant  Value=pos_ki
  Kp : Constant  Value=pos_kp
  Minus : Sum  Inputs=|+-
  Product3 : Product
  Product4 : Product
  Product5 : Product
  Sum : Sum  Inputs=+++|
  torque : Outport
  wires:
  pos_cmd/1 -> Minus/1
  vel/1 -> Gain/1
  Gain/1 -> Product5/2
  Sum/1 -> torque/1
  Product3/1 -> Sum/1
  Kd/1 -> Product5/1
  Minus/1 -> Integrator1/1, Product3/2
  pos/1 -> Minus/2
  Integrator1/1 -> Product4/2
  Kp/1 -> Product3/1
  Ki/1 -> Product4/1
  Product5/1 -> Sum/3
  Product4/1 -> Sum/2

== stateflow chart hexapod_LC/Planner/planner ==
  state Next_step
    entry:
    index=index+1;
    error=inf;
    velx=data1(1,index);
    vely=data1(2,index);
    during:
    dx=wtps(1,index)-statex(1);
    dy=wtps(2, index)-statey;
    posx=wtps(1,index);
    posy= wtps(2,index);
    error=sqrt(dx^2+dy^2);
  state Indexing
    entry:
    number=data;
    index=0;
    velx=data1(1,1);
    vely=data1(2,1);
    posx=startPose(1);
    posy=startPose(2);
    during:
  state End
    entry:
    index=number;
    error=inf;
    velx=0;
    vely=0;
    posx=goalPose(1);
    posy=goalPose(2);
    during:
  (default) -> Indexing
  Next_step -> Next_step [order 1] : [index<number && error<0.4]
  Indexing -> Next_step
  Next_step -> End [order 2] : [index==number && error<0.4]
  data: startPose input; goalPose input; dx local; dy local; error local; data input; number local; index local; data1 input; wtps input; statex input; statey input; vely output; velx output; posy output; posx output
